simulink model "led_switch_logic_simple"  (R2025a)
settings: Solver=FixedStepDiscrete  StartTime=0.0  StopTime=20  FixedStep=1  RelTol=1e-3
libraries: simulink x3
settings Model: Creator=mahij  LastModifiedBy=mahij

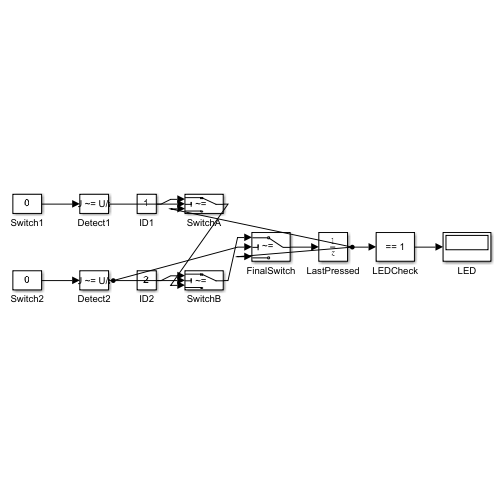
[thumbnail: Simulink's stored preview of the top-level diagram]
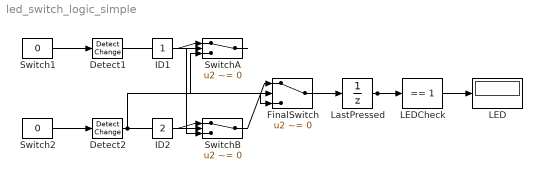
== system led_switch_logic_simple ==
  Detect1 : simulink/Logic and Bit Operations/Detect Change  vinit=0  OutDataTypeStr=boolean
  Detect2 : simulink/Logic and Bit Operations/Detect Change  vinit=0  OutDataTypeStr=boolean
  FinalSwitch : Switch  Criteria=u2 ~= 0  Threshold=0.5  SaturateOnIntegerOverflow=off  InputSameDT=off
  ID1 : Constant
  ID2 : Constant  Value=2
  LED : Display
  LEDCheck : simulink/Logic and Bit Operations/Compare To Constant  relop===  const=1  OutDataTypeStr=boolean
  LastPressed : UnitDelay  HasFrameUpgradeWarning=on
  Switch1 : Constant  Value=0
  Switch2 : Constant  Value=0
  SwitchA : Switch  Criteria=u2 ~= 0  Threshold=0.5  SaturateOnIntegerOverflow=off  InputSameDT=off
  SwitchB : Switch  Criteria=u2 ~= 0  Threshold=0.5  SaturateOnIntegerOverflow=off  InputSameDT=off
  wires:
  Switch1/1 -> Detect1/1
  Switch2/1 -> Detect2/1
  ID1/1 -> SwitchA/1
  Detect1/1 -> SwitchA/2
  LastPressed/1 -> SwitchA/3, FinalSwitch/3, LEDCheck/1
  ID2/1 -> SwitchB/1
  Detect2/1 -> SwitchB/2, FinalSwitch/2
  SwitchA/1 -> SwitchB/3
  SwitchB/1 -> FinalSwitch/1
  FinalSwitch/1 -> LastPressed/1
  LEDCheck/1 -> LED/1
